simulink model "d_loads"  (Simulink 5.1)
settings: Solver=ode45  StartTime=0.0  StopTime=10.0  RelTol=1e-3
settings Model: Creator=fmilano  LastModifiedBy=fmilano  SignalLoggingName=logsout  BooleanDataType=on  RTWOptions="-aEnforceIntegerDowncast=1 -aFoldNonRolledExpr=1 -aInlineInvariantSignals=0 -aInlineParameters=0 -aLocalBlockOutputs=1 -aRollThreshold=5 -aZeroInternalMemoryAtStartup=1 -aZeroExternalMemoryAtStartup=1 -aInitFltsAndDblsToZero=0 -aForceBlockIOInitOptimize=0 -aGenerateReport=0 -aGenCodeOnly=0 -aRTWVerbose=1 -aIncludeHyperlinkInReport=0 -aLaunchReport=0 -aGenerateTraceInfo=0  -aForceParamTrailComments=0 -aGenerateComments=1 -aIgnoreCustomStorageClasses=1 -aIncHierarchyInIds=0 -aMaxRTWIdLen=31 -aShowEliminatedStatements=0 -aIncDataTypeInIds=0 -aInsertBlockDesc=0 -aIgnoreTestpoints=0 -aSimulinkBlockComments=1 -aInlinedPrmAccess=\"Literals\"  -aSuppressErrorStatus=0 -aModelReferenceCompliant=1 -aParenthesesLevel=\"Nominal\" -aModelStepFunctionPrototypeControlCompliant=0 -aPortableWordSizes=0 -aParMdlRefBuildCompliant=1 -aSupportNonInlinedSFcns=1 -aSupportContinuousTime=1 -aSupportComplex=1 -aSupportNonFinite=1 -aSupportAbsoluteTime=1 -aMultiwordLength=2048 -aTargetPreCompLibLocation=\"\" -aTargetLibSuffix=\"\" -aTargetFunctionLibrary=\"ANSI_C\" -aTargetFcnLib=\"ansi_tfl_tmw.mat\" -aMultiInstanceERTCode=0 -aLogVarNameModifier=\"rt_\" -aERTFirstTimeCompliant=0 -aIsPILTarget=0 -aCombineOutputUpdateFcns=0 -aGenerateASAP2=0 -aGenerateClassInterface=0 -aGenerateTestInterfaces=0 -aGenerateSampleERTMain=0 -aGenerateFullHeader=1 -aUtilityFuncGeneration=\"Auto\" -aIncludeFileDelimiter=\"Auto\" -aIncludeMdlTerminateFcn=1 -aPurelyIntegerCode=0 -aAutosarCompliant=0 -aERTCustomFileBanners=0 -aRTWCAPIStates=0 -aRTWCAPIParams=0 -aRTWCAPISignals=0 -aMatFileLogging=1 -aCompOptLevelCompliant=1 -aCPPClassGenCompliant=0 -aExtModeIntrfLevel=\"Level1\" -aExtModeMexFile=\"ext_comm\" -aExtModeTransport=0 -aExtModeStaticAllocSize=1000000 -aExtModeTesting=0 -aExtModeStaticAlloc=0 -aExtMode=0 -aERTMultiwordLength=256 -aERTMultiwordTypeDef=\"System defined\""

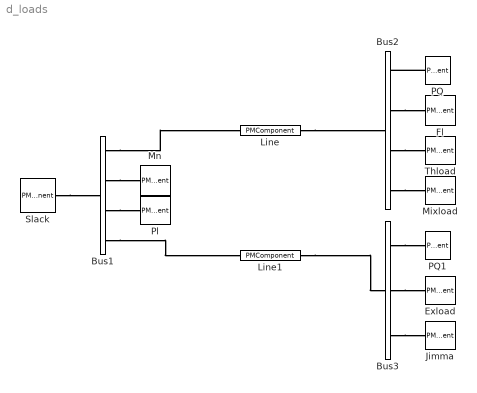
== system d_loads ==
  Bus1 : PMComponent  Tag=PSATblock  Description=Connection  PhysicalDomain=psatdomain  LeftPortType=p1  RightPortType=p1  LConnTagsString=__newl0  RConnTagsString=__newr0|__newr1|__newr2|__newr3  mask(Bus){in=1, out=4, p2q=400, p3_4q=[1.00   0.00], p5q=1, p6q=1}
      mask prompts: in "Number of inputs:"; out "Number of outputs:"; p2q "Voltage Rating [kV]"; p3_4q "Voltage initial guess [p.u.   rad]"; p5q "Area number"; p6q "Region number"
      mask help: Bus block
      mask init:
      | fm_inout
      mask CallbackString: ||||fm_block|
      mask Display: plot([0 1 1 0 0],[0 0 1 1 0])
  Bus2 : PMComponent  Tag=PSATblock  Description=Connection  PhysicalDomain=psatdomain  LeftPortType=p1  RightPortType=p1  LConnTagsString=__newl0  RConnTagsString=__newr0|__newr1|__newr2|__newr3  mask(Bus){in=1, out=4, p2q=400, p3_4q=[1.00   0.00], p5q=1, p6q=1}
      mask prompts: in "Number of inputs:"; out "Number of outputs:"; p2q "Voltage Rating [kV]"; p3_4q "Voltage initial guess [p.u.   rad]"; p5q "Area number"; p6q "Region number"
      mask help: Bus block
      mask init:
      | fm_inout
      mask CallbackString: ||||fm_block|
      mask Display: plot([0 1 1 0 0],[0 0 1 1 0])
  Bus3 : PMComponent  Tag=PSATblock  Description=Connection  PhysicalDomain=psatdomain  LeftPortType=p1  RightPortType=p1  LConnTagsString=__newl0  RConnTagsString=__newr0|__newr1|__newr2  mask(Bus){in=1, out=3, p2q=400, p3_4q=[1.00   0.00], p5q=1, p6q=1}
      mask prompts: in "Number of inputs:"; out "Number of outputs:"; p2q "Voltage Rating [kV]"; p3_4q "Voltage initial guess [p.u.   rad]"; p5q "Area number"; p6q "Region number"
      mask help: Bus block
      mask init:
      | fm_inout
      mask CallbackString: ||||fm_block|
      mask Display: plot([0 1 1 0 0],[0 0 1 1 0])
  Exload : PMComponent  Tag=PSATblock  Description=Loads  PhysicalDomain=psatdomain  LeftPortType=p1  RightPortType=p1  LConnTagsString=__newl0  mask(Exload){p2q=100, p3_4q=[40 40], p5_6q=[1  1], p7_8q=[2   1.5], p9_10q=[2  1.5], p11q=on}
      mask prompts: p2q "Power ratings [MVA]"; p3_4q "Active and reactive power percentages [%, %]"; p5_6q "Time constants for the real and reactive power dynamics Tp, Tq [s, s]"; p7_8q "Real power exponents Alpha_S, Alpha_T"; p9_10q "Reactive power exponents Beta_S, Beta_T"; p11q "Connected"
      mask help: This block defines Exponential Recovery Loads.
      mask init:
      | [x,y] = fm_draw('R');
      mask CallbackString: |||||fm_block
      mask Display:
      | plot([1 0 0 1 1],[1 1 0 0 1])
      | color('blue')
      | plot(0.7+0.3*x,0.6*y+0.5,[0.4 0.1 0.1 0.4],[0.8 0.8 0.2 0.2],[0.1 0.25],[0.5 0.5])
  Fl : PMComponent  Tag=PSATblock  Description=Loads  PhysicalDomain=psatdomain  LeftPortType=p1  RightPortType=p1  LConnTagsString=__newl0  mask(Fl){p2q=30, p3_4q=[2  1.3], p5q=80, p6_7q=[2  1.3], p8q=0.01, p9q=on}
      mask prompts: p2q "Active power percentage Kp [%]"; p3_4q "Active power voltage and frequency exponents ap, bp"; p5q "Reactive power percentage Kq [%]"; p6_7q "Reactive power voltage and frequency exponents aq, bq"; p8q "Frequency filter time constant Tf [s]"; p9q "Connected"
      mask help:
      | This block defines a general exponential voltage
      | frequency dependent load
      mask CallbackString: |||||fm_block
      mask Display:
      | plot([-1 -1 1 1 -1],[-1 1 1 -1 -1])
      | color('blue')
      | plot([-0.2 -0.15 0 0 0.15 0.2],[-0.45 -0.5 -0.4 0.35 0.45 0.35],[-0.1 0.15],[0.05 0.05])
  Jimma : PMComponent  Tag=PSATblock  Description=Loads  PhysicalDomain=psatdomain  LeftPortType=p1  RightPortType=p1  LConnTagsString=__newl0  mask(Jimma){p2_3_4q=[100  400  60], p6_7_8q=[20 20 20], p9_10_11q=[20 20 20], p5q=0.01, p12q=100, p13q=on}
      mask prompts: p2_3_4q "Power, voltage and frequency ratings [MVA, kV, Hz]"; p6_7_8q "Percentage of resistance, active current and active power [% % %]"; p9_10_11q "Percentage of reactance, reactive current and reactive power [% % %]"; p5q "High-pass filter time constant Tf [s]"; p12q "Coefficient of voltage time derivative KV [1/s]"; p13q "Connected"
      mask help: This block defines a Jimma's Load.
      mask init:
      | [x,y] = fm_draw('J');
      mask CallbackString: |||||fm_block
      mask Display:
      | plot([-1 -1 1 1 -1],[-1 1 1 -1 -1]);
      | color('blue')
      | plot(x,y)
  Line : PMComponent  Tag=PSATblock  Description=Power Flow  PhysicalDomain=psatdomain  LeftPortType=p1  RightPortType=p1  LConnTagsString=__newl0  RConnTagsString=__newr0  mask(Line){p3_4_5q=[100  400  60], p6q=0, p8q=0.01, p9q=0.10, p10q=1e-3, p13_14_15q=[0.0  0.0  0.0], p16q=on}
      mask prompts: p3_4_5q "Power, Voltage and Frequency Ratings [MVA, kV, Hz]"; p6q "Length of line [km] (0 for p.u. parameters)"; p8q "Resistance [p.u. (Ohms/km)]"; p9q "Reactance [p.u. (H/km)]"; p10q "Susceptance [p.u. (F/km)]"; p13_14_15q "Imax, Pmax and Smax [p.u., p.u., p.u.]"; p16q "Connected"
      mask help: This block defines a pi model for a tree phase line.
      mask init:
      | [xp,yp] = fm_draw('pi');
      mask CallbackString: ||||||fm_block
      mask Display:
      | plot([-1  1  1 -1 -1],[-0.2 -0.2 0.2 0.2 -0.2])
      | color('blue')
      | plot(0.35*xp,0.2*yp)
  Line1 : PMComponent  Tag=PSATblock  Description=Power Flow  PhysicalDomain=psatdomain  LeftPortType=p1  RightPortType=p1  LConnTagsString=__newl0  RConnTagsString=__newr0  mask(Line){p3_4_5q=[100  400  60], p6q=0, p8q=0.01, p9q=0.10, p10q=1e-3, p13_14_15q=[0.0  0.0  0.0], p16q=on}
      mask prompts: p3_4_5q "Power, Voltage and Frequency Ratings [MVA, kV, Hz]"; p6q "Length of line [km] (0 for p.u. parameters)"; p8q "Resistance [p.u. (Ohms/km)]"; p9q "Reactance [p.u. (H/km)]"; p10q "Susceptance [p.u. (F/km)]"; p13_14_15q "Imax, Pmax and Smax [p.u., p.u., p.u.]"; p16q "Connected"
      mask help: This block defines a pi model for a tree phase line.
      mask init:
      | [xp,yp] = fm_draw('pi');
      mask CallbackString: ||||||fm_block
      mask Display:
      | plot([-1  1  1 -1 -1],[-0.2 -0.2 0.2 0.2 -0.2])
      | color('blue')
      | plot(0.35*xp,0.2*yp)
  Mixload : PMComponent  Tag=PSATblock  Description=Loads  PhysicalDomain=psatdomain  LeftPortType=p1  RightPortType=p1  LConnTagsString=__newl0  mask(Mixload){p2_3_4q=[100  400  60], p6_10q=[20 20], p5_9q=[0  0], p7_11q=[0  0], p8_12q=[0.12  0.075], p13_14q=[0.005  0.007], p15q=on}
      mask prompts: p2_3_4q "Power, voltage and frequency ratings [MVA, kV, Hz]"; p6_10q "Percentage of active and reactive power Kpv and Kqv [% %]"; p5_9q "Frequency coefficients Kpf and Kqf"; p7_11q "Voltage exponents alpha and beta"; p8_12q "Time constant of dV/dt Tpv and Tqv [s s]"; p13_14q "Filter time constants Tfv and Tft [s s]"; p15q "Connected"
      mask help: This block defines a mixed load.
      mask CallbackString: ||||||fm_block
      mask Display:
      | plot([-1 -1 2.4 2.4 -1],[-1 1 1 -1 -1])
      | color('blue')
      | plot([-0.35 -0.35 0 0.35 0.35],[-0.35 0.35 0.05 0.35 -0.35])
      | plot([0.7 0.7],[-0.35 0.35])
      | plot([1.05 1.75],[-0.35 0.35],[1.05 1.75],[0.35 -0.35])
  Mn : PMComponent  Tag=PSATblock  Description=Loads  PhysicalDomain=psatdomain  LeftPortType=p1  RightPortType=p1  LConnTagsString=__newl0  mask(Mn){p2_3q=[100 400], p4_5q=[0.8  0.6], p6_7q=[2.00 2.00], p8q=off, p9q=on}
      mask prompts: p2_3q "Power and voltage ratings [MVA, kV]"; p4_5q "Active && reactive powers [p.u., p.u.]"; p6_7q "Voltage exponents for the active and reactive powers"; p8q "Initialize after power flow"; p9q "Connected"
      mask help: This block defines a general exponential voltage load.
      mask CallbackString: |||fm_block|fm_block
      mask Display:
      | plot([-1 -1 1 1 -1],[-1 1 1 -1 -1])
      | color('blue')
      | plot([-0.35 -0.35 0 0.35 0.35],[-0.35 0.35 0.05 0.35 -0.35])
  PQ : PMComponent  Tag=PSATblock  Description=Power Flow  PhysicalDomain=psatdomain  LeftPortType=p1  RightPortType=p1  LConnTagsString=__newl0  mask(PQ){p2_3q=[100  400], p4_5q=[0.80  0.60], p6_7q=[1.2  0.8], p8q=on, p9q=on}
      mask prompts: p2_3q "Power and Voltage Ratings [MVA, kV]"; p4_5q "Active and Reactive Powers [p.u.  p.u.]"; p6_7q "Maximum and Minimum Allowable Voltage [p.u.   p.u.]"; p8q "Allow conversion to impendance for min or max voltage"; p9q "Connected"
      mask help:
      | This block defines a constant power load:
      |
      | P = Pcost.
      | Q = Qcost.
      mask CallbackString: |||fm_block|fm_block
      mask Display: plot([1 -0.5 -0.5 1],[0 0.866 -0.866 0])
  PQ1 : PMComponent  Tag=PSATblock  Description=Power Flow  PhysicalDomain=psatdomain  LeftPortType=p1  RightPortType=p1  LConnTagsString=__newl0  mask(PQ){p2_3q=[100  400], p4_5q=[0.80  0.60], p6_7q=[1.2  0.8], p8q=on, p9q=on}
      mask prompts: p2_3q "Power and Voltage Ratings [MVA, kV]"; p4_5q "Active and Reactive Powers [p.u.  p.u.]"; p6_7q "Maximum and Minimum Allowable Voltage [p.u.   p.u.]"; p8q "Allow conversion to impendance for min or max voltage"; p9q "Connected"
      mask help:
      | This block defines a constant power load:
      |
      | P = Pcost.
      | Q = Qcost.
      mask CallbackString: |||fm_block|fm_block
      mask Display: plot([1 -0.5 -0.5 1],[0 0.866 -0.866 0])
  Pl : PMComponent  Tag=PSATblock  Description=Loads  PhysicalDomain=psatdomain  LeftPortType=p1  RightPortType=p1  LConnTagsString=__newl0  mask(Pl){p2_3_4q=[100 400 60], p5_6_7q=[0.33 0.33 0.33], p8_9_10q=[0.33 0.33 0.33], p11q=off, p12q=on}
      mask prompts: p2_3_4q "Power, voltage and frequency ratings [MVA, kV, Hz]"; p5_6_7q "Resistance, active current and active power [p.u., p.u., p.u.]"; p8_9_10q "Reactance, reactive current and reactive power [p.u., p.u., p.u.]"; p11q "Initialize after power flow"; p12q "Connected"
      mask help: This block defines a ZIP load.
      mask CallbackString: |||fm_block|fm_block
      mask Display:
      | plot([-1 -1 1 1 -1],[-1 1 1 -1 -1])
      | color('blue')
      | plot([0 0],[-0.3 0.3],[-0.3 -0.7 -0.3 -0.7],[-0.3 -0.3 0.3 0.3])
      | plot([0.3 0.3 0.6 0.7 0.7 0.6 0.3],[-0.3 0.3 0.3 0.2 0.1 0 0])
  Slack : PMComponent  Tag=PSATblock  Description=Power Flow  PhysicalDomain=psatdomain  LeftPortType=p1  RightPortType=p1  RConnTagsString=__newr0  mask(SW){p2_3q=[100  400], p4q=1.00, p5q=0.00, p6_7q=[1.5  -1.5], p8_9q=[1.1  0.9], p10q=0.80, p11q=1, p12q=on, p13q=on}
      mask prompts: p2_3q "Power and Voltage Ratings [MVA, kV]"; p4q "Voltage Magnitude [p.u.]"; p5q "Reference Phase Angle [rad]"; p6_7q "Qmax and Qmin [p.u.  p.u.]"; p8_9q "Vmax and Vmin  [p.u.  p.u.]"; p10q "Active Power Guess [p.u.]"; p11q "Loss Participation Factor"; p12q "Reference bus"; p13q "Connected"
      mask help:
      | This block defines a V-theta bus:
      |
      | V = V_des
      | theta = theta_des
      mask init:
      | [x,y] = fm_draw('circle');
      | [xt,yt] = fm_draw('theta');
      mask CallbackString: |||||||fm_block|fm_block
      mask Display: plot([0 1 1 0 0],[0 0 1 1 0]), color('blue'), plot([0 1],[0 1],[0 1],[1 0],[0.5 1 0.5 0 0.5],[0 0.5 1 0.5 0])
  Thload : PMComponent  Tag=PSATblock  Description=Loads  PhysicalDomain=psatdomain  LeftPortType=p1  RightPortType=p1  LConnTagsString=__newl0  mask(Thload){p2q=50, p3q=100, p4q=25, p5q=10, p6q=1200, p7q=10, p8q=70, p11q=2, p12q=on}
      mask prompts: p2q "% of load to be used as thermostatically controlled load [%]"; p3q "Gain of proportional controller Kp"; p4q "Gain of integral controller Ki"; p5q "Time constant of integral controller Ti [s]"; p6q "Thermostatically controlled load time constant T1 [s]"; p7q "Ambient temperature Ta [F]"; p8q "Reference temperature Tref [F]"; p11q "Ceiling conductance ouput KL"; p12q "Connected"
      mask help: This block defines a thermostatically controlled load
      mask CallbackString: ||||||||fm_block
      mask Display:
      | plot([-1 -1 1 1 -1],[-1 1 1 -1 -1])
      | color('blue')
      | plot([-0.5 -0.5 -0.25 -0.25 -0.5],[0.4 0.15 0.15 0.4 0.4])
      | plot([-0.05 -0.05 0.5],[-0.4 0.4 0.4],[-0.05 0.3],[0.05 0.05])
  connections:
  Slack/RConn1 -- Bus1/LConn1
  Line/RConn1 -- Bus2/LConn1
  PQ/LConn1 -- Bus2/RConn1
  Bus2/RConn2 -- Fl/LConn1
  Bus1/RConn3 -- Pl/LConn1
  Bus1/RConn4 -- Line1/LConn1
  Line1/RConn1 -- Bus3/LConn1
  Bus3/RConn1 -- PQ1/LConn1
  Bus3/RConn2 -- Exload/LConn1
  Bus1/RConn2 -- Mn/LConn1
  Bus1/RConn1 -- Line/LConn1
  Bus2/RConn3 -- Thload/LConn1
  Bus3/RConn3 -- Jimma/LConn1
  Bus2/RConn4 -- Mixload/LConn1
